simulink model "controller"  (R2018b)
settings: Solver=VariableStepAuto  StartTime=0.0  StopTime=10.0  RelTol=1e-3
settings Model: Creator=jayakumarav  LastModifiedBy=hiterd
settings DebuggingCC: LibraryContextMissingDiagnostic=none
settings SFSimCC: SimUseLocalCustomCode=off
settings RTWCC: RTWUseLocalCustomCode=off

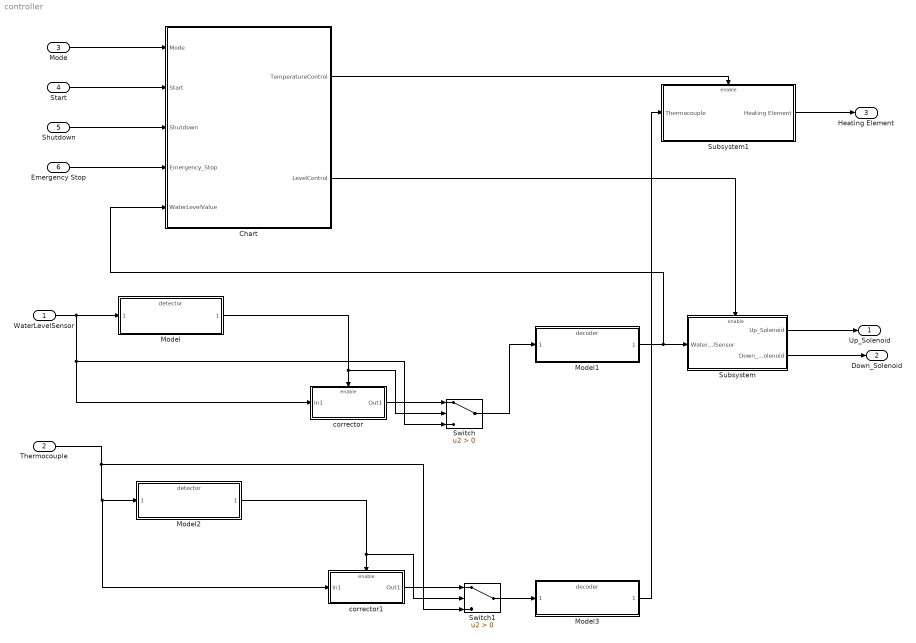
== system controller ==
  WaterLevelSensor : Inport
  Thermocouple : Inport  Port=2
  Mode : Inport  Port=3
  Start : Inport  Port=4
  Shutdown : Inport  Port=5
  Emergency Stop : Inport  Port=6
  Chart : Stateflow chart  TreatAsAtomicUnit=on
  Model : ModelReference  ModelNameDialog=detector.slx  SimulationMode=Normal  ModelReferenceVersion=1.21
  Model1 : ModelReference  ModelNameDialog=decoder.slx  SimulationMode=Normal  ModelReferenceVersion=1.22
  Model2 : ModelReference  ModelNameDialog=detector.slx  SimulationMode=Normal  ModelReferenceVersion=1.21
  Model3 : ModelReference  ModelNameDialog=decoder.slx  SimulationMode=Normal  ModelReferenceVersion=1.22
  Subsystem : Subsystem
  Subsystem1 : Subsystem
  Switch : Switch  Criteria=u2 > Threshold
  Switch1 : Switch  Criteria=u2 > Threshold
  corrector : Subsystem
  corrector1 : Subsystem
  Up_Solenoid : Outport
  Down_Solenoid : Outport  Port=2
  Heating Element : Outport  Port=3
  wires:
  Mode/1 -> Chart/1(Mode)
  Chart/2(LevelControl) -> Subsystem/Enable
  Chart/1(TemperatureControl) -> Subsystem1/Enable
  Emergency Stop/1 -> Chart/4(Emergency_Stop)
  Subsystem1/1(Heating Element) -> Heating Element/1
  Shutdown/1 -> Chart/3(Shutdown)
  Start/1 -> Chart/2(Start)
  Subsystem/2(Down_Solenoid) -> Down_Solenoid/1
  Subsystem/1(Up_Solenoid) -> Up_Solenoid/1
  Model/1 -> corrector/Enable, Switch/2
  corrector/1(Out1) -> Switch/1
  WaterLevelSensor/1 -> Switch/3, corrector/1(In1), Model/1
  Switch/1 -> Model1/1
  Model1/1 -> Chart/5(WaterLevelValue), Subsystem/1(WaterLevelSensor)
  corrector1/1(Out1) -> Switch1/1
  Switch1/1 -> Model3/1
  Model2/1 -> corrector1/Enable, Switch1/2
  Thermocouple/1 -> Switch1/3, corrector1/1(In1), Model2/1
  Model3/1 -> Subsystem1/1(Thermocouple)

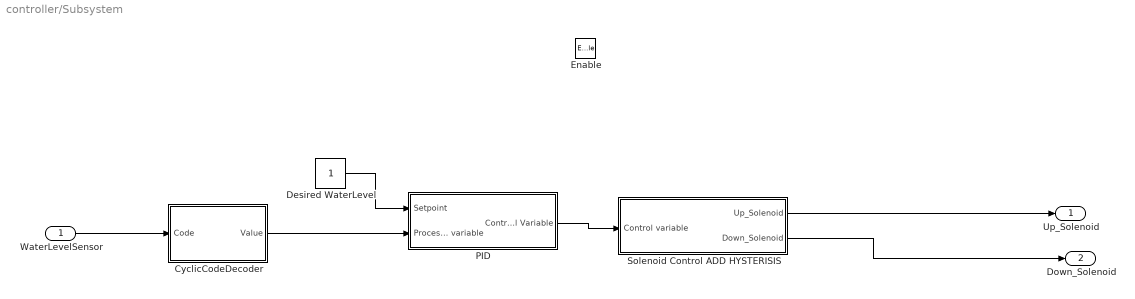
== system controller/Subsystem ==
  WaterLevelSensor : Inport
  Enable : EnablePort
  CyclicCodeDecoder : Subsystem  TreatAsAtomicUnit=on
  Desired WaterLevel : Constant
  PID : Subsystem  TreatAsAtomicUnit=on
  Solenoid Control ADD HYSTERISIS : Subsystem  TreatAsAtomicUnit=on
  Up_Solenoid : Outport
  Down_Solenoid : Outport  Port=2
  wires:
  Solenoid Control ADD HYSTERISIS/2(Down_Solenoid) -> Down_Solenoid/1
  PID/1(Control Variable) -> Solenoid Control ADD HYSTERISIS/1(Control variable)
  CyclicCodeDecoder/1(Value) -> PID/2(Process variable)
  Solenoid Control ADD HYSTERISIS/1(Up_Solenoid) -> Up_Solenoid/1
  Desired WaterLevel/1 -> PID/1(Setpoint)
  WaterLevelSensor/1 -> CyclicCodeDecoder/1(Code)

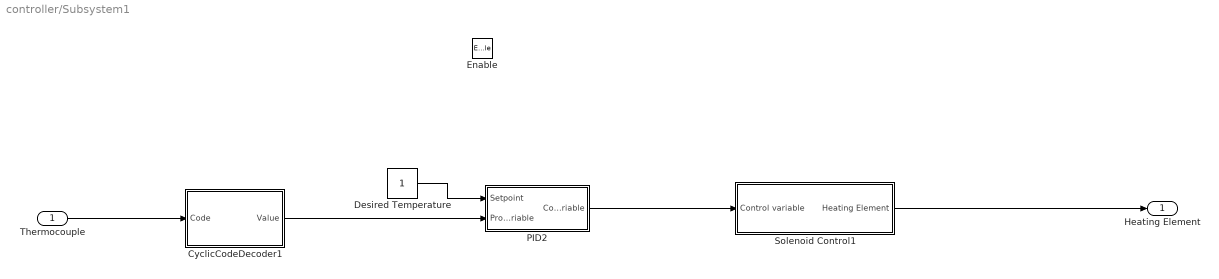
== system controller/Subsystem1 ==
  Thermocouple : Inport
  Enable : EnablePort
  CyclicCodeDecoder1 : Subsystem  TreatAsAtomicUnit=on
  Desired Temperature : Constant
  PID2 : Subsystem  TreatAsAtomicUnit=on
  Solenoid Control1 : Subsystem  TreatAsAtomicUnit=on
  Heating Element : Outport
  wires:
  Thermocouple/1 -> CyclicCodeDecoder1/1(Code)
  Solenoid Control1/1(Heating Element) -> Heating Element/1
  Desired Temperature/1 -> PID2/1(Setpoint)
  CyclicCodeDecoder1/1(Value) -> PID2/2(Process variable)
  PID2/1(Control Variable) -> Solenoid Control1/1(Control variable)

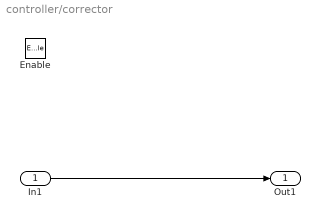
== system controller/corrector ==
  In1 : Inport
  Enable : EnablePort
  Out1 : Outport
  wires:
  In1/1 -> Out1/1

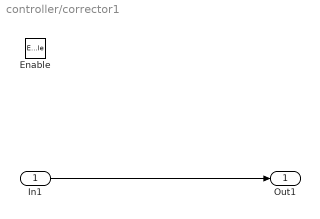
== system controller/corrector1 ==
  In1 : Inport
  Enable : EnablePort
  Out1 : Outport
  wires:
  In1/1 -> Out1/1

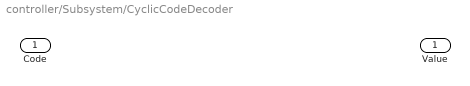
== system controller/Subsystem/CyclicCodeDecoder ==
  Code : Inport
  Value : Outport

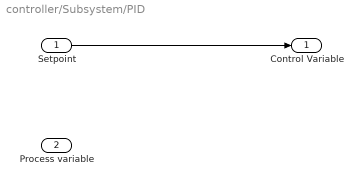
== system controller/Subsystem/PID ==
  Setpoint : Inport
  Process variable : Inport  Port=2
  Control Variable : Outport
  wires:
  Setpoint/1 -> Control Variable/1

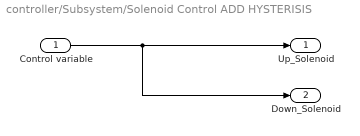
== system controller/Subsystem/Solenoid Control ADD HYSTERISIS ==
  Control variable : Inport
  Up_Solenoid : Outport
  Down_Solenoid : Outport  Port=2
  wires:
  Control variable/1 -> Down_Solenoid/1, Up_Solenoid/1

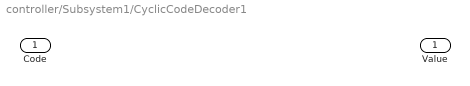
== system controller/Subsystem1/CyclicCodeDecoder1 ==
  Code : Inport
  Value : Outport

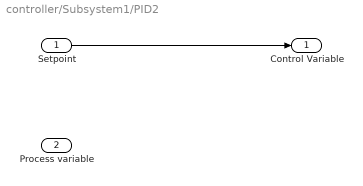
== system controller/Subsystem1/PID2 ==
  Setpoint : Inport
  Process variable : Inport  Port=2
  Control Variable : Outport
  wires:
  Setpoint/1 -> Control Variable/1

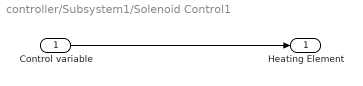
== system controller/Subsystem1/Solenoid Control1 ==
  Control variable : Inport
  Heating Element : Outport
  wires:
  Control variable/1 -> Heating Element/1

== stateflow chart controller/Chart ==
  data: TemperatureControl output; Mode input; Start input; Shutdown input; Emergency_Stop input; WaterLevelValue input; LevelControl output
